simulink library "lib_ofdmrx"  (R2020a)
settings: Solver=VariableStepAuto  StartTime=0.0  StopTime=10.0  RelTol=1e-3
undefined symbols (not defined in the file): fs, LTSfreq, pilot, read_addr_rx, sc_index
libraries: simulink x36, hdlsllib x28, dspsigops x4, dsphdlmathfun x3, dsphdlxfrm x1, dsphdlsigops x1
(part 1 of 3)
settings Model: Creator=LDM  LastModifiedBy=LDM

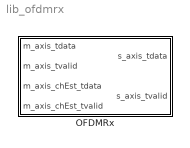
== system lib_ofdmrx ==
  OFDMRx : Subsystem  TreatAsAtomicUnit=on

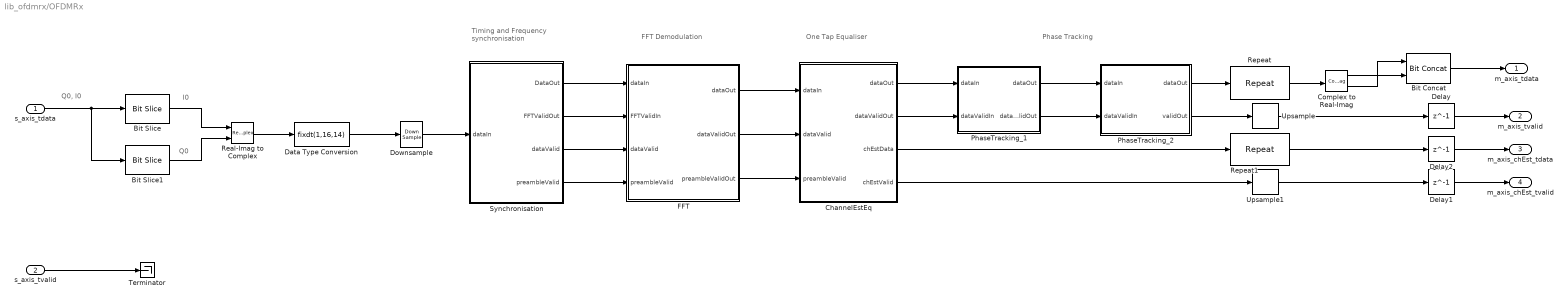
== system lib_ofdmrx/OFDMRx ==
  note: Q0
  note: I0
  note: Q0, I0
  note: Timing and Frequency
      | synchronisation
  note: FFT Demodulation
  note: One Tap Equaliser
  note: Phase Tracking
  s_axis_tdata : Inport
  s_axis_tvalid : Inport  Port=2
  Bit Concat : hdlsllib/Logic and Bit Operations/Bit Concat  numInputs=2
  Bit Slice : hdlsllib/Logic and Bit Operations/Bit Slice  lidx=15  ridx=0
      settings: SourceProductBaseCode=SL
  Bit Slice1 : hdlsllib/Logic and Bit Operations/Bit Slice  lidx=31  ridx=16
      settings: SourceProductBaseCode=SL
  ChannelEstEq : Subsystem
  Complex to Real-Imag : ComplexToRealImag
  Data Type Conversion : DataTypeConversion  OutDataTypeStr=fixdt(1,16,14)  ConvertRealWorld=Stored Integer (SI)
  Delay : Delay  DelayLength=1
  Delay1 : Delay  DelayLength=1
  Delay2 : Delay  DelayLength=1
  Downsample : DownSample  N=12  RateOptions=Allow multirate processing
  FFT : Subsystem
  PhaseTracking_1 : Subsystem
  PhaseTracking_2 : Subsystem
  Real-Imag to Complex : RealImagToComplex
  Repeat : dspsigops/Repeat  N=12  InputProcessing=Columns as channels (frame based)  RateOptions=Allow multirate processing  ic=0  mode=Unused parameter value
  Repeat1 : dspsigops/Repeat  N=12  InputProcessing=Columns as channels (frame based)  RateOptions=Allow multirate processing  ic=0  mode=Unused parameter value
  Synchronisation : Subsystem
  Terminator : Terminator
  Upsample : dspsigops/Upsample  N=12  phase=5  RateOptions=Allow multirate processing  ic=0  mode=Unused parameter value
  Upsample1 : dspsigops/Upsample  N=12  phase=5  RateOptions=Allow multirate processing  ic=0  mode=Unused parameter value
  m_axis_tdata : Outport  VectorParamsAs1DForOutWhenUnconnected=off
  m_axis_tvalid : Outport  Port=2  VectorParamsAs1DForOutWhenUnconnected=off
  m_axis_chEst_tdata : Outport  Port=3  VectorParamsAs1DForOutWhenUnconnected=off
  m_axis_chEst_tvalid : Outport  Port=4  VectorParamsAs1DForOutWhenUnconnected=off
  wires:
  Delay2/1 -> m_axis_chEst_tdata/1
  Repeat1/1 -> Delay2/1
  ChannelEstEq/3(chEstData) -> Repeat1/1
  ChannelEstEq/4(chEstValid) -> Upsample1/1
  Delay1/1 -> m_axis_chEst_tvalid/1
  Upsample1/1 -> Delay1/1
  PhaseTracking_1/2(dataValidOut) -> PhaseTracking_2/2(dataValidIn)
  PhaseTracking_1/1(dataOut) -> PhaseTracking_2/1(dataIn)
  ChannelEstEq/2(dataValidOut) -> PhaseTracking_1/2(dataValidIn)
  ChannelEstEq/1(dataOut) -> PhaseTracking_1/1(dataIn)
  Synchronisation/4(preambleValid) -> FFT/4(preambleValid)
  Synchronisation/3(dataValid) -> FFT/3(dataValid)
  Synchronisation/2(FFTValidOut) -> FFT/2(FFTValidIn)
  Synchronisation/1(DataOut) -> FFT/1(dataIn)
  FFT/2(dataValidOut) -> ChannelEstEq/2(dataValid)
  FFT/3(preambleValidOut) -> ChannelEstEq/3(preambleValid)
  FFT/1(dataOut) -> ChannelEstEq/1(dataIn)
  Real-Imag to Complex/1 -> Data Type Conversion/1
  Downsample/1 -> Synchronisation/1(dataIn)
  PhaseTracking_2/1(dataOut) -> Repeat/1
  PhaseTracking_2/2(validOut) -> Upsample/1
  Repeat/1 -> Complex to Real-Imag/1
  Complex to Real-Imag/2 -> Bit Concat/1
  Complex to Real-Imag/1 -> Bit Concat/2
  Bit Concat/1 -> m_axis_tdata/1
  Bit Slice/1 -> Real-Imag to Complex/1
  Bit Slice1/1 -> Real-Imag to Complex/2
  s_axis_tdata/1 -> Bit Slice1/1, Bit Slice/1
  s_axis_tvalid/1 -> Terminator/1
  Data Type Conversion/1 -> Downsample/1
  Upsample/1 -> Delay/1
  Delay/1 -> m_axis_tvalid/1

== system lib_ofdmrx/OFDMRx/ChannelEstEq ==
  dataIn : Inport
  dataValid : Inport  Port=2
  preambleValid : Inport  Port=3
  Bit Concat1 : hdlsllib/Logic and Bit Operations/Bit Concat  numInputs=2
  ChannelEstimate : Subsystem
  Complex to Real-Imag1 : ComplexToRealImag
  Data Type Conversion1 : DataTypeConversion  OutDataTypeStr=fixdt(1,16,14)
  Data Type Conversion3 : DataTypeConversion  OutDataTypeStr=uint16  ConvertRealWorld=Stored Integer (SI)
  Data Type Conversion4 : DataTypeConversion  OutDataTypeStr=uint16  ConvertRealWorld=Stored Integer (SI)
  Delay : Delay  DelayLength=6
  Equalise : Subsystem
  dataOut : Outport  VectorParamsAs1DForOutWhenUnconnected=off
  dataValidOut : Outport  Port=2  VectorParamsAs1DForOutWhenUnconnected=off
  chEstData : Outport  Port=3  VectorParamsAs1DForOutWhenUnconnected=off
  chEstValid : Outport  Port=4  VectorParamsAs1DForOutWhenUnconnected=off
  wires:
  Data Type Conversion1/1 -> Complex to Real-Imag1/1
  Complex to Real-Imag1/1 -> Data Type Conversion3/1
  Complex to Real-Imag1/2 -> Data Type Conversion4/1
  Data Type Conversion3/1 -> Bit Concat1/2
  Bit Concat1/1 -> chEstData/1
  Data Type Conversion4/1 -> Bit Concat1/1
  ChannelEstimate/2(dataValidOut) -> Equalise/3(dataValidIn), chEstValid/1
  Equalise/2(dataValidOut) -> dataValidOut/1
  Equalise/1(dataOutEq) -> dataOut/1
  dataValid/1 -> ChannelEstimate/3(dataValidIn)
  preambleValid/1 -> ChannelEstimate/2(preambleValid)
  dataIn/1 -> Delay/1, ChannelEstimate/1(dataIn)
  Delay/1 -> Equalise/1(dataInEq)
  ChannelEstimate/1(chEstOut) -> Data Type Conversion1/1, Equalise/2(chEstIn)

== system lib_ofdmrx/OFDMRx/FFT ==
  dataIn : Inport
  FFTValidIn : Inport  Port=2
  dataValid : Inport  Port=3
  preambleValid : Inport  Port=4
  Delay1 : Delay  DelayLength=173
  Delay2 : Delay  DelayLength=173
  FFT HDL Optimized : dsphdlxfrm/FFT HDL Optimized  FFTLength=64  Architecture=Streaming Radix 2^2  ComplexMultiplication=Use 4 multipliers and 2 adders  BitReversedOutput=off  BitReversedInput=off  Normalize=off  SimulateUsing=Code generation  RoundingMethod=Floor  ResetInputPort=off  StartOutputPort=off  EndOutputPort=off
      settings: SourceProductBaseCode=DS
  Terminator : Terminator
  dataOut : Outport  VectorParamsAs1DForOutWhenUnconnected=off
  dataValidOut : Outport  Port=2  VectorParamsAs1DForOutWhenUnconnected=off
  preambleValidOut : Outport  Port=3  VectorParamsAs1DForOutWhenUnconnected=off
  wires:
  preambleValid/1 -> Delay1/1
  dataValid/1 -> Delay2/1
  FFT HDL Optimized/2 -> Terminator/1
  FFT HDL Optimized/1 -> dataOut/1
  Delay1/1 -> preambleValidOut/1
  Delay2/1 -> dataValidOut/1
  dataIn/1 -> FFT HDL Optimized/1
  FFTValidIn/1 -> FFT HDL Optimized/2

== system lib_ofdmrx/OFDMRx/PhaseTracking_1 ==
  note: Phase Tracking Stage 1: Track linear phase error which occurs due to sampling phase/frequency offsets. The implemented algorithm
      | estimates the gradient of the linear phase error using pilot sub-carriers.
  dataIn : Inport
  dataValidIn : Inport  Port=2
  CordicRotate : Subsystem
  DataArrange : Subsystem
  "GradientEstimate " : Subsystem
  PhaseErrorEst : Subsystem
  PilotCtrlGen : Subsystem
  dataOut : Outport
  dataValidOut : Outport  Port=2
  wires:
  PilotCtrlGen/4(dataValid) -> "GradientEstimate "/4(dataValid)
  PilotCtrlGen/3(pilotEnd) -> "GradientEstimate "/3(PilotEnd)
  PilotCtrlGen/2(pilotOut) -> "GradientEstimate "/2(pilotIn)
  PilotCtrlGen/1(dataOut) -> "GradientEstimate "/1(dataIn)
  DataArrange/2(dataValidOut) -> PilotCtrlGen/2(validIn)
  DataArrange/1(dataOut) -> PilotCtrlGen/1(dataIn)
  dataValidIn/1 -> DataArrange/2(dataValidIn)
  dataIn/1 -> DataArrange/1(dataIn)
  CordicRotate/1("DataOutRotate  ") -> dataOut/1
  "GradientEstimate "/3(dataValidOut) -> PhaseErrorEst/3(dataValidIn)
  "GradientEstimate "/2(gradientOut) -> PhaseErrorEst/2(gradientIn)
  "GradientEstimate "/1(dataOut) -> PhaseErrorEst/1(dataIn)
  PhaseErrorEst/1(dataOut) -> CordicRotate/1(DataInRotate)
  PhaseErrorEst/2(PhaseOut) -> CordicRotate/2(PhaseInRotate)
  PhaseErrorEst/3(dataValidOut) -> CordicRotate/3(dataValidIn)
  CordicRotate/2(dataValidOut) -> dataValidOut/1

== system lib_ofdmrx/OFDMRx/PhaseTracking_2 ==
  note: Phase Tracking Stage 2:  Track Common Phase Error (CPE) from symbol to symbol.
      | CPE is caused by residual frequency offset and phase noise effects.
  dataIn : Inport
  dataValidIn : Inport  Port=2
  CordicRotate : Subsystem
  PhaseEst : Subsystem
  PilotCtrlGen : Subsystem
  dataOut : Outport  VectorParamsAs1DForOutWhenUnconnected=off
  validOut : Outport  Port=2  VectorParamsAs1DForOutWhenUnconnected=off
  wires:
  dataValidIn/1 -> PilotCtrlGen/2(ValidIn)
  dataIn/1 -> PilotCtrlGen/1(dataIn)
  CordicRotate/2(validOut) -> validOut/1
  CordicRotate/1("DataOut  ") -> dataOut/1
  PhaseEst/3(validOut) -> CordicRotate/3(validIn)
  PhaseEst/2(phaseOut) -> CordicRotate/2(PhaseIn)
  PhaseEst/1(dataOut) -> CordicRotate/1(DataIn)
  PilotCtrlGen/4(dataValid) -> PhaseEst/4(dataValid)
  PilotCtrlGen/3(PilotEnd) -> PhaseEst/3(pilotEnd)
  PilotCtrlGen/2(pilotOut) -> PhaseEst/2(PilotIn)
  PilotCtrlGen/1(dataOut) -> PhaseEst/1(dataIn)

== system lib_ofdmrx/OFDMRx/Synchronisation ==
  dataIn : Inport
  CoarseFreqCorr : Subsystem
  ControlSigGen : Subsystem
  Delay : Subsystem
  Delay1 : Delay  DelayLength=22  InputProcessing=Columns as channels (frame based)
  Delay2 : Delay  InputProcessing=Columns as channels (frame based)
  Delay4 : Delay  DelayLength=1  InputProcessing=Columns as channels (frame based)
  FrameDetect : Subsystem
  "SchmidlCoxMetric " : Subsystem
  DataOut : Outport  VectorParamsAs1DForOutWhenUnconnected=off
  FFTValidOut : Outport  Port=2  VectorParamsAs1DForOutWhenUnconnected=off
  dataValid : Outport  Port=3  VectorParamsAs1DForOutWhenUnconnected=off
  preambleValid : Outport  Port=4  VectorParamsAs1DForOutWhenUnconnected=off
  wires:
  Delay/1(dataOut) -> Delay4/1
  Delay/2(strobeOut) -> ControlSigGen/1(validIn)
  CoarseFreqCorr/1(dataOut) -> Delay/1(data)
  CoarseFreqCorr/2(frameDetOut) -> Delay/2(strobe)
  Delay4/1 -> DataOut/1
  FrameDetect/1(frameDet) -> CoarseFreqCorr/2(frameDet)
  Delay2/1 -> CoarseFreqCorr/1(dataIn)
  FrameDetect/2(phaseOut) -> CoarseFreqCorr/3(phaseIn)
  "SchmidlCoxMetric "/3(phase) -> FrameDetect/3(phaseIn)
  "SchmidlCoxMetric "/2(right) -> FrameDetect/2(rightIn)
  "SchmidlCoxMetric "/1(left) -> FrameDetect/1(leftIn)
  Delay1/1 -> Delay2/1
  ControlSigGen/3(preambleValid) -> preambleValid/1
  ControlSigGen/2(dataValid) -> dataValid/1
  ControlSigGen/1(FFTValid) -> FFTValidOut/1
  dataIn/1 -> Delay1/1, "SchmidlCoxMetric "/1(dataIn)

== system lib_ofdmrx/OFDMRx/ChannelEstEq/ChannelEstimate ==
  note: Get and store the channel estimate using the two
      | repetitions of the L-LTF
  note: Write averaged channel estimate to RAM and read out when data is valid
      | for equalisation of successive OFDM symbols.
  note: Note the preamble symbols do not pass this point.
  dataIn : Inport
  preambleValid : Inport  Port=2
  dataValidIn : Inport  Port=3
  ChanEst : Subsystem
  Delay : Delay  DelayLength=5
  Delay1 : Delay  DelayLength=5
  Delay2 : Delay  DelayLength=1
  Dual Port RAM1 : hdlsllib/HDL RAMs/Dual Port RAM  ram_size=6
      settings: SourceProductBaseCode=SL
  HDL Counter3 : hdlsllib/Sources/HDL Counter  CountType=Count limited  CountInit=0  CountStep=1  CountMax=63  CountFromType=Initial value  CountFrom=0  CountResetPort=off  CountLoadPort=off  CountEnbPort=on  CountDirPort=off  CountDataType=Unsigned  CountWordLen=6  CountFracLen=0  CountSampTime=1
  Terminator : Terminator
  WriteEnbAddrGen : Subsystem
  chEstOut : Outport  VectorParamsAs1DForOutWhenUnconnected=off
  dataValidOut : Outport  Port=2  VectorParamsAs1DForOutWhenUnconnected=off
  wires:
  Dual Port RAM1/1 -> Terminator/1
  WriteEnbAddrGen/2(Out2) -> Dual Port RAM1/3
  WriteEnbAddrGen/1(Out1) -> Dual Port RAM1/2
  Delay/1 -> WriteEnbAddrGen/1(In1)
  Delay1/1 -> Delay2/1, HDL Counter3/1
  dataValidIn/1 -> Delay1/1
  ChanEst/1(ChEstOut) -> Dual Port RAM1/1
  dataIn/1 -> ChanEst/1(ChanEstIn)
  preambleValid/1 -> Delay/1, ChanEst/2(PreambValidIn)
  Delay2/1 -> dataValidOut/1
  Dual Port RAM1/2 -> chEstOut/1
  HDL Counter3/1 -> Dual Port RAM1/4

== system lib_ofdmrx/OFDMRx/ChannelEstEq/Equalise ==
  note: Perform a complex division to obtain equalised data symbols.
  dataInEq : Inport
  chEstIn : Inport  Port=2
  dataValidIn : Inport  Port=3
  Abs2 : Subsystem
  Complex Mult : Subsystem
  Delay1 : Delay
  Delay8 : Delay  DelayLength=3
  Divide : Subsystem
  dataOutEq : Outport  VectorParamsAs1DForOutWhenUnconnected=off
  dataValidOut : Outport  Port=2  VectorParamsAs1DForOutWhenUnconnected=off
  wires:
  Divide/1(dataOutEq) -> dataOutEq/1
  Delay1/1 -> dataValidOut/1
  Delay8/1 -> Delay1/1
  Abs2/1(Out1) -> Divide/2(In2)
  Complex Mult/1(Out1) -> Divide/1(In1)
  dataInEq/1 -> Complex Mult/1(In1)
  chEstIn/1 -> Complex Mult/2(In2), Abs2/1(ChEstIn)
  dataValidIn/1 -> Delay8/1

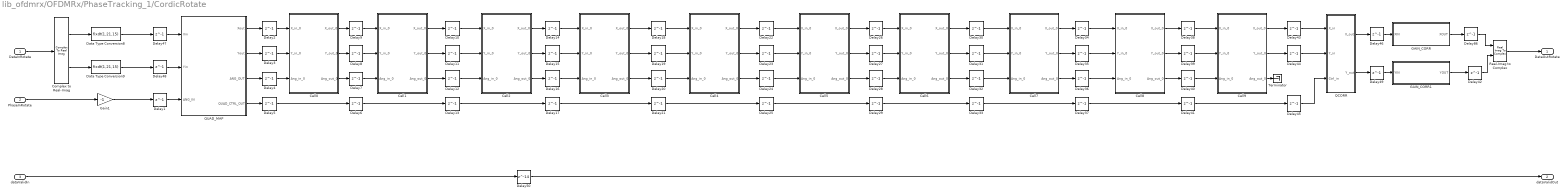
== system lib_ofdmrx/OFDMRx/PhaseTracking_1/CordicRotate ==
  DataInRotate : Inport
  PhaseInRotate : Inport  Port=2
  dataValidIn : Inport  Port=3
  Cell0 : Subsystem
  Cell1 : Subsystem
  Cell2 : Subsystem
  Cell3 : Subsystem
  Cell4 : Subsystem
  Cell5 : Subsystem
  Cell6 : Subsystem
  Cell7 : Subsystem
  Cell8 : Subsystem
  Cell9 : Subsystem
  Complex to Real-Imag : ComplexToRealImag
  Data Type Conversion8 : DataTypeConversion  OutDataTypeStr=fixdt(1,21,15)
  Data Type Conversion9 : DataTypeConversion  OutDataTypeStr=fixdt(1,21,15)
  Delay{1..49,86} (50 alike) : Delay  DelayLength=1
  Delay50 : Delay  DelayLength=14
  GAIN_CORR : Subsystem
  GAIN_CORR1 : Subsystem
  Gain1 : Gain  Gain=-1  OutDataTypeStr=fixdt(1,23,20)
  QCORR : Subsystem
  QUAD_MAP : Subsystem
  Real-Imag to Complex : RealImagToComplex
  Terminator : Terminator
  "DataOutRotate  " : Outport  VectorParamsAs1DForOutWhenUnconnected=off
  dataValidOut : Outport  Port=2  VectorParamsAs1DForOutWhenUnconnected=off
  wires:
  Real-Imag to Complex/1 -> "DataOutRotate  "/1
  Delay42/1 -> Real-Imag to Complex/2
  Delay86/1 -> Real-Imag to Complex/1
  Complex to Real-Imag/1 -> Data Type Conversion8/1
  DataInRotate/1 -> Complex to Real-Imag/1
  Complex to Real-Imag/2 -> Data Type Conversion9/1
  GAIN_CORR/1(XOUT) -> Delay86/1
  Delay48/1 -> QUAD_MAP/2(Yin)
  Delay47/1 -> QUAD_MAP/1(Xin)
  QUAD_MAP/1(Xout) -> Delay2/1
  QUAD_MAP/2(Yout) -> Delay3/1
  QUAD_MAP/3(ANG_OUT) -> Delay4/1
  Delay2/1 -> Cell0/1(X_in_0)
  Delay3/1 -> Cell0/2(Y_in_0)
  QUAD_MAP/4(QUAD_CTRL_OUT) -> Delay5/1
  Cell0/1(X_out_0) -> Delay9/1
  Cell0/2(Y_out_0) -> Delay8/1
  Cell0/3(Ang_out_0) -> Delay7/1
  Delay5/1 -> Delay6/1
  Delay7/1 -> Cell1/3(Ang_in_0)
  Delay8/1 -> Cell1/2(Y_in_0)
  Delay9/1 -> Cell1/1(X_in_0)
  Cell1/1(X_out_0) -> Delay10/1
  Cell1/2(Y_out_0) -> Delay11/1
  Cell1/3(Ang_out_0) -> Delay12/1
  Delay6/1 -> Delay13/1
  Delay10/1 -> Cell2/1(X_in_0)
  Delay11/1 -> Cell2/2(Y_in_0)
  Delay12/1 -> Cell2/3(Ang_in_0)
  Delay16/1 -> Cell3/3(Ang_in_0)
  Delay15/1 -> Cell3/2(Y_in_0)
  Delay14/1 -> Cell3/1(X_in_0)
  Delay13/1 -> Delay17/1
  Cell2/3(Ang_out_0) -> Delay16/1
  Cell2/2(Y_out_0) -> Delay15/1
  Cell2/1(X_out_0) -> Delay14/1
  Cell3/1(X_out_0) -> Delay18/1
  Cell3/2(Y_out_0) -> Delay19/1
  Cell3/3(Ang_out_0) -> Delay20/1
  Delay17/1 -> Delay21/1
  Delay18/1 -> Cell4/1(X_in_0)
  Delay19/1 -> Cell4/2(Y_in_0)
  Delay20/1 -> Cell4/3(Ang_in_0)
  Delay24/1 -> Cell5/3(Ang_in_0)
  Delay23/1 -> Cell5/2(Y_in_0)
  Delay22/1 -> Cell5/1(X_in_0)
  Delay21/1 -> Delay25/1
  Cell4/3(Ang_out_0) -> Delay24/1
  Cell4/2(Y_out_0) -> Delay23/1
  Cell4/1(X_out_0) -> Delay22/1
  Cell5/1(X_out_0) -> Delay26/1
  Cell5/2(Y_out_0) -> Delay27/1
  Cell5/3(Ang_out_0) -> Delay28/1
  Delay25/1 -> Delay29/1
  Delay26/1 -> Cell6/1(X_in_0)
  Delay27/1 -> Cell6/2(Y_in_0)
  Delay28/1 -> Cell6/3(Ang_in_0)
  Delay32/1 -> Cell7/3(Ang_in_0)
  Delay31/1 -> Cell7/2(Y_in_0)
  Delay30/1 -> Cell7/1(X_in_0)
  Delay29/1 -> Delay33/1
  Cell6/3(Ang_out_0) -> Delay32/1
  Cell6/2(Y_out_0) -> Delay31/1
  Cell6/1(X_out_0) -> Delay30/1
  Cell7/1(X_out_0) -> Delay34/1
  Cell7/2(Y_out_0) -> Delay35/1
  Cell7/3(Ang_out_0) -> Delay36/1
  Delay33/1 -> Delay37/1
  Delay34/1 -> Cell8/1(X_in_0)
  Delay35/1 -> Cell8/2(Y_in_0)
  Delay36/1 -> Cell8/3(Ang_in_0)
  Delay40/1 -> Cell9/3(Ang_in_0)
  Delay39/1 -> Cell9/2(Y_in_0)
  Delay38/1 -> Cell9/1(X_in_0)
  Delay37/1 -> Delay41/1
  Cell8/3(Ang_out_0) -> Delay40/1
  Cell8/2(Y_out_0) -> Delay39/1
  Cell8/1(X_out_0) -> Delay38/1
  GAIN_CORR1/1(YOUT) -> Delay42/1
  Cell9/3(Ang_out_0) -> Terminator/1
  Delay41/1 -> Delay45/1
  Cell9/1(X_out_0) -> Delay43/1
  Cell9/2(Y_out_0) -> Delay44/1
  Delay43/1 -> QCORR/1(X_in)
  Delay44/1 -> QCORR/2(Y_in)
  Delay46/1 -> GAIN_CORR/1(XIN)
  Delay49/1 -> GAIN_CORR1/1(YIN)
  QCORR/2(Y_out) -> Delay49/1
  Delay1/1 -> QUAD_MAP/3(ANG_IN)
  Delay4/1 -> Cell0/3(Ang_in_0)
  Delay45/1 -> QCORR/3(Ctrl_in)
  Data Type Conversion8/1 -> Delay47/1
  Data Type Conversion9/1 -> Delay48/1
  QCORR/1(X_out) -> Delay46/1
  PhaseInRotate/1 -> Gain1/1
  Gain1/1 -> Delay1/1
  dataValidIn/1 -> Delay50/1
  Delay50/1 -> dataValidOut/1

== system lib_ofdmrx/OFDMRx/PhaseTracking_1/DataArrange ==
  note: Re-arrange data symbols
  dataIn : Inport
  dataValidIn : Inport  Port=2
  Delay : Delay  DelayLength=64  InitialCondition=0  UseCircularBuffer=on
  Delay3 : Delay  DelayLength=1  InitialCondition=0  UseCircularBuffer=on
  Dual Port RAM : hdlsllib/HDL RAMs/Dual Port RAM  ram_size=7
      settings: SourceProductBaseCode=SL
  HDL Counter : hdlsllib/Sources/HDL Counter  CountType=Count limited  CountInit=0  CountStep=1  CountMax=127  CountFromType=Initial value  CountFrom=0  CountResetPort=off  CountLoadPort=off  CountEnbPort=on  CountDirPort=off  CountDataType=Unsigned  CountWordLen=7  CountFracLen=0  CountSampTime=1
  HDL Counter1 : hdlsllib/Sources/HDL Counter  CountType=Count limited  CountInit=0  CountStep=1  CountMax=127  CountFromType=Initial value  CountFrom=0  CountResetPort=off  CountLoadPort=off  CountEnbPort=on  CountDirPort=off  CountDataType=Unsigned  CountWordLen=7  CountFracLen=0  CountSampTime=1
  READ_ADDRESS : Lookup_n-D  NumberOfTableDimensions=1  LookupTableObject=''  BreakpointsForDimension1=[0:127]  BreakpointsForDimension1FirstPoint=10  BreakpointsForDimension2FirstPoint=10  BreakpointsForDimension1Spacing=12  BreakpointsForDimension2Spacing=12  IndexSearchMethod=Evenly spaced points  Table=read_addr_rx  TableDataTypeStr=fixdt(0,7,0)  InterpMethod=Flat  DiagnosticForOutOfRangeInput=Error  InternalRulePriority=Speed  OutDataTypeStr=fixdt(0,7,0)  RndMeth=Simplest  InputSameDT=on
  READ_CTRL : Subsystem
  Terminator : Terminator
  dataValidGen : Subsystem
  dataOut : Outport  VectorParamsAs1DForOutWhenUnconnected=off
  dataValidOut : Outport  Port=2  VectorParamsAs1DForOutWhenUnconnected=off
  wires:
  dataValidGen/1(dataValidOut) -> dataValidOut/1
  Delay3/1 -> dataValidGen/1(enb)
  READ_ADDRESS/1 -> READ_CTRL/1(In1)
  READ_CTRL/1(Out1) -> Dual Port RAM/4
  Delay/1 -> READ_CTRL/2(In2), Delay3/1, HDL Counter/1
  HDL Counter1/1 -> Dual Port RAM/2
  dataIn/1 -> Dual Port RAM/1
  Dual Port RAM/2 -> dataOut/1
  HDL Counter/1 -> READ_ADDRESS/1
  dataValidIn/1 -> Dual Port RAM/3, HDL Counter1/1, Delay/1
  Dual Port RAM/1 -> Terminator/1

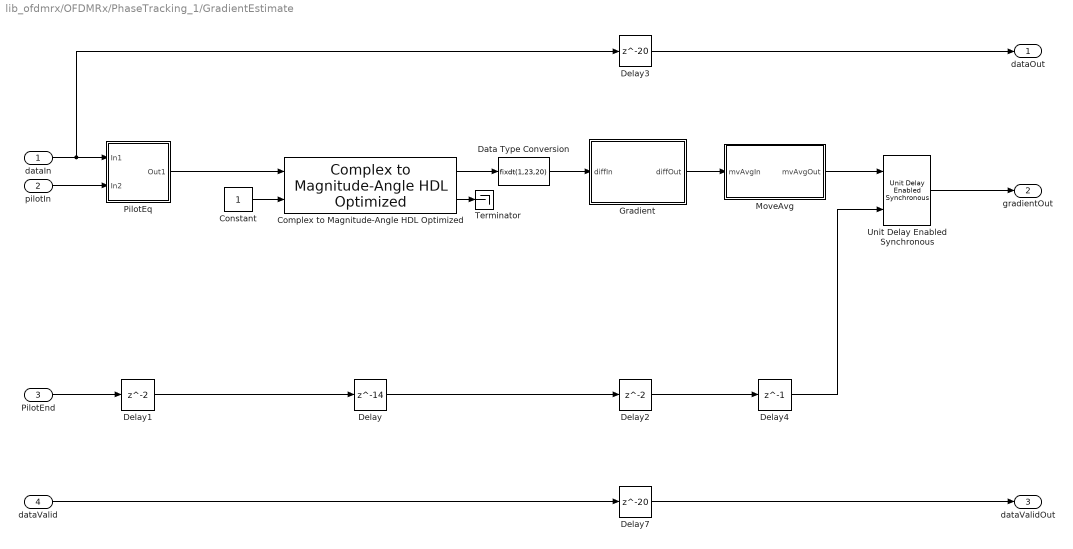
== system lib_ofdmrx/OFDMRx/PhaseTracking_1/GradientEstimate  ==
  dataIn : Inport
  pilotIn : Inport  Port=2
  PilotEnd : Inport  Port=3
  dataValid : Inport  Port=4
  Complex to Magnitude-Angle HDL Optimized : dsphdlmathfun/Complex to Magnitude-Angle HDL Optimized  NumIterationsSource=Property  NumIterations=10  OutputFormat=Angle  AngleFormat=Radians  ScaleOutput=off  SimulateUsing=Code generation
      settings: SourceProductBaseCode=DS
  Constant : Constant  OutDataTypeStr=boolean  SampleTime=1/fs
  Data Type Conversion : DataTypeConversion  OutDataTypeStr=fixdt(1,23,20)
  Delay : Delay  DelayLength=14
  Delay1 : Delay
  Delay2 : Delay
  Delay3 : Delay  DelayLength=20
  Delay4 : Delay  DelayLength=1
  Delay7 : Delay  DelayLength=20
  Gradient : Subsystem
  MoveAvg : Subsystem
  PilotEq : Subsystem
  Terminator : Terminator
  Unit Delay Enabled Synchronous : hdlsllib/Discrete/Unit Delay Enabled Synchronous  InitialCondition=0.0  SampleTime=-1
      settings: SourceProductBaseCode=SL
  dataOut : Outport  VectorParamsAs1DForOutWhenUnconnected=off
  gradientOut : Outport  Port=2  VectorParamsAs1DForOutWhenUnconnected=off
  dataValidOut : Outport  Port=3  VectorParamsAs1DForOutWhenUnconnected=off
  wires:
  Delay4/1 -> Unit Delay Enabled Synchronous/2
  Delay/1 -> Delay2/1
  PilotEnd/1 -> Delay1/1
  dataValid/1 -> Delay7/1
  Gradient/1(diffOut) -> MoveAvg/1(mvAvgIn)
  dataIn/1 -> Delay3/1, PilotEq/1(In1)
  pilotIn/1 -> PilotEq/2(In2)
  PilotEq/1(Out1) -> Complex to Magnitude-Angle HDL Optimized/1
  Delay1/1 -> Delay/1
  MoveAvg/1(mvAvgOut) -> Unit Delay Enabled Synchronous/1
  Delay3/1 -> dataOut/1
  Unit Delay Enabled Synchronous/1 -> gradientOut/1
  Delay7/1 -> dataValidOut/1
  Complex to Magnitude-Angle HDL Optimized/1 -> Data Type Conversion/1
  Constant/1 -> Complex to Magnitude-Angle HDL Optimized/2
  Complex to Magnitude-Angle HDL Optimized/2 -> Terminator/1
  Data Type Conversion/1 -> Gradient/1(diffIn)
  Delay2/1 -> Delay4/1

== system lib_ofdmrx/OFDMRx/PhaseTracking_1/PhaseErrorEst ==
  dataIn : Inport
  gradientIn : Inport  Port=2
  dataValidIn : Inport  Port=3
  Delay{2..8} (7 alike) : Delay  DelayLength=1
  HDL Counter : hdlsllib/Sources/HDL Counter  CountType=Count limited  CountInit=0  CountStep=1  CountMax=51  CountFromType=Initial value  CountFrom=0  CountResetPort=on  CountLoadPort=off  CountEnbPort=on  CountDirPort=off  CountDataType=Unsigned  CountWordLen=6  CountFracLen=0  CountSampTime=1
  LUT : Lookup_n-D  NumberOfTableDimensions=1  BreakpointsForDimension1=0:51  IndexSearchMethod=Evenly spaced points  Table=sc_index  TableDataTypeStr=fixdt(1,6,0)  InterpMethod=Flat  ExtrapMethod=Clip  DiagnosticForOutOfRangeInput=Error  UseLastTableValue=on  InternalRulePriority=Speed  OutDataTypeStr=fixdt(1,6,0)  RndMeth=Simplest  InputSameDT=on
  NOT : Logic  Operator=NOT  IconShape=distinctive  AllPortsSameDT=off  OutDataTypeStr=boolean
  Product : Product  OutDataTypeStr=fixdt(1,23,20)
  dataOut : Outport  VectorParamsAs1DForOutWhenUnconnected=off
  PhaseOut : Outport  Port=2  VectorParamsAs1DForOutWhenUnconnected=off
  dataValidOut : Outport  Port=3  VectorParamsAs1DForOutWhenUnconnected=off
  wires:
  dataValidIn/1 -> NOT/1, Delay4/1, HDL Counter/2
  dataIn/1 -> Delay2/1
  gradientIn/1 -> Delay3/1
  LUT/1 -> Delay5/1
  NOT/1 -> HDL Counter/1
  HDL Counter/1 -> LUT/1
  Delay3/1 -> Product/1
  Delay5/1 -> Product/2
  Delay2/1 -> Delay6/1
  Delay6/1 -> dataOut/1
  Product/1 -> Delay7/1
  Delay7/1 -> PhaseOut/1
  Delay4/1 -> Delay8/1
  Delay8/1 -> dataValidOut/1

== system lib_ofdmrx/OFDMRx/PhaseTracking_1/PilotCtrlGen ==
  dataIn : Inport
  validIn : Inport  Port=2
  CtrlSigGen : Subsystem
  Delay1 : Delay  DelayLength=1
  Delay10 : Delay  DelayLength=1
  SampleCounter : Subsystem
  SymbolCounter : Subsystem
  pilotGen : Subsystem
  dataOut : Outport  VectorParamsAs1DForOutWhenUnconnected=off
  pilotOut : Outport  Port=2  VectorParamsAs1DForOutWhenUnconnected=off
  pilotEnd : Outport  Port=3  VectorParamsAs1DForOutWhenUnconnected=off
  dataValid : Outport  Port=4  VectorParamsAs1DForOutWhenUnconnected=off
  wires:
  Delay1/1 -> pilotGen/3(valid), CtrlSigGen/1(valid)
  SampleCounter/1(Sample_Cnt) -> pilotGen/2(sampleCount), CtrlSigGen/2(sampleCount)
  CtrlSigGen/2(pilotEnd) -> pilotEnd/1
  CtrlSigGen/1(dataValid) -> dataValid/1
  SymbolCounter/1(Symbl_cnt) -> pilotGen/1(symbCount)
  validIn/1 -> Delay1/1, SampleCounter/1(Valid_In), SymbolCounter/1(ValidIn)
  pilotGen/1(pilOut) -> pilotOut/1
  Delay10/1 -> dataOut/1
  dataIn/1 -> Delay10/1

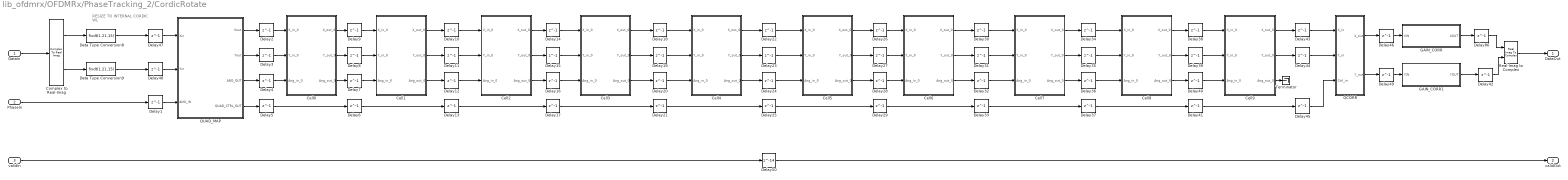
== system lib_ofdmrx/OFDMRx/PhaseTracking_2/CordicRotate ==
  note: RESIZE TO INTERNAL
      | CORDIC WL
  DataIn : Inport
  PhaseIn : Inport  Port=2
  validIn : Inport  Port=3
  Cell0 : Subsystem
  Cell1 : Subsystem
  Cell2 : Subsystem
  Cell3 : Subsystem
  Cell4 : Subsystem
  Cell5 : Subsystem
  Cell6 : Subsystem
  Cell7 : Subsystem
  Cell8 : Subsystem
  Cell9 : Subsystem
  Complex to Real-Imag : ComplexToRealImag
  Data Type Conversion8 : DataTypeConversion  OutDataTypeStr=fixdt(1,21,15)
  Data Type Conversion9 : DataTypeConversion  OutDataTypeStr=fixdt(1,21,15)
  Delay{1..49,86} (50 alike) : Delay  DelayLength=1
  Delay50 : Delay  DelayLength=14
  GAIN_CORR : Subsystem
  GAIN_CORR1 : Subsystem
  QCORR : Subsystem
  QUAD_MAP : Subsystem
  Real-Imag to Complex : RealImagToComplex
  Terminator : Terminator
  "DataOut  " : Outport  VectorParamsAs1DForOutWhenUnconnected=off
  validOut : Outport  Port=2  VectorParamsAs1DForOutWhenUnconnected=off
  wires:
  Delay50/1 -> validOut/1
  validIn/1 -> Delay50/1
  Real-Imag to Complex/1 -> "DataOut  "/1
  Delay42/1 -> Real-Imag to Complex/2
  Delay86/1 -> Real-Imag to Complex/1
  Complex to Real-Imag/1 -> Data Type Conversion8/1
  DataIn/1 -> Complex to Real-Imag/1
  Complex to Real-Imag/2 -> Data Type Conversion9/1
  GAIN_CORR/1(XOUT) -> Delay86/1
  Delay48/1 -> QUAD_MAP/2(Yin)
  Delay47/1 -> QUAD_MAP/1(Xin)
  QUAD_MAP/1(Xout) -> Delay2/1
  QUAD_MAP/2(Yout) -> Delay3/1
  QUAD_MAP/3(ANG_OUT) -> Delay4/1
  Delay2/1 -> Cell0/1(X_in_0)
  Delay3/1 -> Cell0/2(Y_in_0)
  QUAD_MAP/4(QUAD_CTRL_OUT) -> Delay5/1
  Cell0/1(X_out_0) -> Delay9/1
  Cell0/2(Y_out_0) -> Delay8/1
  Cell0/3(Ang_out_0) -> Delay7/1
  Delay5/1 -> Delay6/1
  Delay7/1 -> Cell1/3(Ang_in_0)
  Delay8/1 -> Cell1/2(Y_in_0)
  Delay9/1 -> Cell1/1(X_in_0)
  Cell1/1(X_out_0) -> Delay10/1
  Cell1/2(Y_out_0) -> Delay11/1
  Cell1/3(Ang_out_0) -> Delay12/1
  Delay6/1 -> Delay13/1
  Delay10/1 -> Cell2/1(X_in_0)
  Delay11/1 -> Cell2/2(Y_in_0)
  Delay12/1 -> Cell2/3(Ang_in_0)
  Delay16/1 -> Cell3/3(Ang_in_0)
  Delay15/1 -> Cell3/2(Y_in_0)
  Delay14/1 -> Cell3/1(X_in_0)
  Delay13/1 -> Delay17/1
  Cell2/3(Ang_out_0) -> Delay16/1
  Cell2/2(Y_out_0) -> Delay15/1
  Cell2/1(X_out_0) -> Delay14/1
  Cell3/1(X_out_0) -> Delay18/1
  Cell3/2(Y_out_0) -> Delay19/1
  Cell3/3(Ang_out_0) -> Delay20/1
  Delay17/1 -> Delay21/1
  Delay18/1 -> Cell4/1(X_in_0)
  Delay19/1 -> Cell4/2(Y_in_0)
  Delay20/1 -> Cell4/3(Ang_in_0)
  Delay24/1 -> Cell5/3(Ang_in_0)
  Delay23/1 -> Cell5/2(Y_in_0)
  Delay22/1 -> Cell5/1(X_in_0)
  Delay21/1 -> Delay25/1
  Cell4/3(Ang_out_0) -> Delay24/1
  Cell4/2(Y_out_0) -> Delay23/1
  Cell4/1(X_out_0) -> Delay22/1
  Cell5/1(X_out_0) -> Delay26/1
  Cell5/2(Y_out_0) -> Delay27/1
  Cell5/3(Ang_out_0) -> Delay28/1
  Delay25/1 -> Delay29/1
  Delay26/1 -> Cell6/1(X_in_0)
  Delay27/1 -> Cell6/2(Y_in_0)
  Delay28/1 -> Cell6/3(Ang_in_0)
  Delay32/1 -> Cell7/3(Ang_in_0)
  Delay31/1 -> Cell7/2(Y_in_0)
  Delay30/1 -> Cell7/1(X_in_0)
  Delay29/1 -> Delay33/1
  Cell6/3(Ang_out_0) -> Delay32/1
  Cell6/2(Y_out_0) -> Delay31/1
  Cell6/1(X_out_0) -> Delay30/1
  Cell7/1(X_out_0) -> Delay34/1
  Cell7/2(Y_out_0) -> Delay35/1
  Cell7/3(Ang_out_0) -> Delay36/1
  Delay33/1 -> Delay37/1
  Delay34/1 -> Cell8/1(X_in_0)
  Delay35/1 -> Cell8/2(Y_in_0)
  Delay36/1 -> Cell8/3(Ang_in_0)
  Delay40/1 -> Cell9/3(Ang_in_0)
  Delay39/1 -> Cell9/2(Y_in_0)
  Delay38/1 -> Cell9/1(X_in_0)
  Delay37/1 -> Delay41/1
  Cell8/3(Ang_out_0) -> Delay40/1
  Cell8/2(Y_out_0) -> Delay39/1
  Cell8/1(X_out_0) -> Delay38/1
  GAIN_CORR1/1(YOUT) -> Delay42/1
  Cell9/3(Ang_out_0) -> Terminator/1
  Delay41/1 -> Delay45/1
  Cell9/1(X_out_0) -> Delay43/1
  Cell9/2(Y_out_0) -> Delay44/1
  Delay43/1 -> QCORR/1(X_in)
  Delay44/1 -> QCORR/2(Y_in)
  Delay46/1 -> GAIN_CORR/1(XIN)
  Delay49/1 -> GAIN_CORR1/1(YIN)
  QCORR/2(Y_out) -> Delay49/1
  Delay1/1 -> QUAD_MAP/3(ANG_IN)
  Delay4/1 -> Cell0/3(Ang_in_0)
  Delay45/1 -> QCORR/3(Ctrl_in)
  Data Type Conversion8/1 -> Delay47/1
  Data Type Conversion9/1 -> Delay48/1
  PhaseIn/1 -> Delay1/1
  QCORR/1(X_out) -> Delay46/1

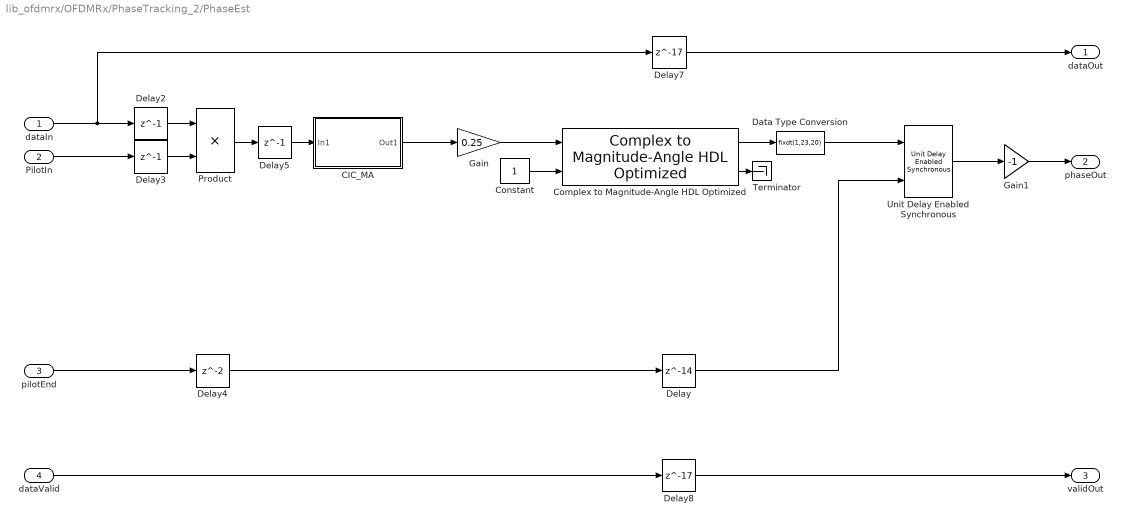
== system lib_ofdmrx/OFDMRx/PhaseTracking_2/PhaseEst ==
  dataIn : Inport
  PilotIn : Inport  Port=2
  pilotEnd : Inport  Port=3
  dataValid : Inport  Port=4
  CIC_MA : Subsystem
  Complex to Magnitude-Angle HDL Optimized : dsphdlmathfun/Complex to Magnitude-Angle HDL Optimized  NumIterationsSource=Property  NumIterations=10  OutputFormat=Angle  AngleFormat=Radians  ScaleOutput=off  SimulateUsing=Code generation
      settings: SourceProductBaseCode=DS
  Constant : Constant  OutDataTypeStr=boolean  SampleTime=1/fs
  Data Type Conversion : DataTypeConversion  OutDataTypeStr=fixdt(1,23,20)
  Delay : Delay  DelayLength=14
  Delay2 : Delay  DelayLength=1
  Delay3 : Delay  DelayLength=1
  Delay4 : Delay
  Delay5 : Delay  DelayLength=1
  Delay7 : Delay  DelayLength=17
  Delay8 : Delay  DelayLength=17
  Gain : Gain  Gain=0.25  OutDataTypeStr=fixdt(1,18,15)
  Gain1 : Gain  Gain=-1  OutDataTypeStr=fixdt(1,23,20)
  Product : Product  OutDataTypeStr=fixdt(1,18,15)
  Terminator : Terminator
  Unit Delay Enabled Synchronous : hdlsllib/Discrete/Unit Delay Enabled Synchronous  InitialCondition=0.0  SampleTime=-1
      settings: SourceProductBaseCode=SL
  dataOut : Outport  VectorParamsAs1DForOutWhenUnconnected=off
  phaseOut : Outport  Port=2  VectorParamsAs1DForOutWhenUnconnected=off
  validOut : Outport  Port=3  VectorParamsAs1DForOutWhenUnconnected=off
  wires:
  Data Type Conversion/1 -> Unit Delay Enabled Synchronous/1
  Gain1/1 -> phaseOut/1
  Delay4/1 -> Delay/1
  Complex to Magnitude-Angle HDL Optimized/2 -> Terminator/1
  Complex to Magnitude-Angle HDL Optimized/1 -> Data Type Conversion/1
  Gain/1 -> Complex to Magnitude-Angle HDL Optimized/1
  Constant/1 -> Complex to Magnitude-Angle HDL Optimized/2
  Delay8/1 -> validOut/1
  Unit Delay Enabled Synchronous/1 -> Gain1/1
  Delay7/1 -> dataOut/1
  dataValid/1 -> Delay8/1
  pilotEnd/1 -> Delay4/1
  Delay5/1 -> CIC_MA/1(In1)
  Delay3/1 -> Product/2
  Delay2/1 -> Product/1
  Product/1 -> Delay5/1
  dataIn/1 -> Delay2/1, Delay7/1
  PilotIn/1 -> Delay3/1
  Delay/1 -> Unit Delay Enabled Synchronous/2
  CIC_MA/1(Out1) -> Gain/1

== system lib_ofdmrx/OFDMRx/PhaseTracking_2/PilotCtrlGen ==
  dataIn : Inport
  ValidIn : Inport  Port=2
  CtrlSigGen : Subsystem
  Delay1 : Delay  DelayLength=1
  Delay10 : Delay  DelayLength=1
  SampleCounter : Subsystem
  SymbolCounter : Subsystem
  pilotGen : Subsystem
  dataOut : Outport  VectorParamsAs1DForOutWhenUnconnected=off
  pilotOut : Outport  Port=2  VectorParamsAs1DForOutWhenUnconnected=off
  PilotEnd : Outport  Port=3  VectorParamsAs1DForOutWhenUnconnected=off
  dataValid : Outport  Port=4  VectorParamsAs1DForOutWhenUnconnected=off
  wires:
  Delay1/1 -> pilotGen/3(valid), CtrlSigGen/1(valid)
  SampleCounter/1(Sample_Cnt) -> pilotGen/2(sampleCount), CtrlSigGen/2(sampleCount)
  CtrlSigGen/2(pilotEnd) -> PilotEnd/1
  CtrlSigGen/1(dataValid) -> dataValid/1
  SymbolCounter/1(Symbl_cnt) -> pilotGen/1(symbCount)
  ValidIn/1 -> SymbolCounter/1(ValidIn), SampleCounter/1(Valid_In), Delay1/1
  pilotGen/1(pilOut) -> pilotOut/1
  Delay10/1 -> dataOut/1
  dataIn/1 -> Delay10/1

== system lib_ofdmrx/OFDMRx/Synchronisation/CoarseFreqCorr ==
  note: Reccord the phase of the averaged autocorrelation at the coarse
      | timing point.
  note: Correct frequency offset
  note: Generate complex sinusoid with a frequency equal
      | to the estimated frequency offset.
  dataIn : Inport
  frameDet : Inport  Port=2
  phaseIn : Inport  Port=3
  Constant : Constant  VectorParams1D=off  OutDataTypeStr=boolean  SampleTime=1/fs
  Delay{,2,5,7} (4 alike) : Delay  DelayLength=1
  Delay1 : Delay  DelayLength=9
  Delay3 : Delay  DelayLength=6
  Gain : Gain  Gain=2048  OutDataTypeStr=uint16
  Math Function : Math  Operator=conj  SignedPower=on  RndMeth=Zero  SaturateOnIntegerOverflow=on
  NCO HDL Optimized : dsphdlsigops/NCO HDL Optimized  PhaseIncrementSource=Input port  PhaseIncrement=100  PhaseOffsetSource=Property  PhaseOffset=0  DitherSource=Property  NumDitherBits=4  SamplesPerFrame=1  LUTCompress=on  ResetAction=off  Waveform=Complex exponential  PhasePort=off  SimulateUsing=Code generation  AccumulatorWL=16  PhaseQuantization=on  NumQuantizerAccumulatorBits=12  OutputDataType=Binary point scaling  OutputWL=16  OutputFL=14
      settings: SourceProductBaseCode=DS
  Product : Product  OutDataTypeStr=fixdt(1,16,14)
  RsingEdge : Subsystem
  Terminator : Terminator
  Unit Delay Enabled Synchronous : hdlsllib/Discrete/Unit Delay Enabled Synchronous  InitialCondition=0.0  SampleTime=-1
      settings: SourceProductBaseCode=SL
  dataOut : Outport  VectorParamsAs1DForOutWhenUnconnected=off
  frameDetOut : Outport  Port=2  VectorParamsAs1DForOutWhenUnconnected=off
  wires:
  Delay7/1 -> dataOut/1
  Delay1/1 -> frameDetOut/1
  Math Function/1 -> Delay5/1
  Delay3/1 -> Delay/1
  Product/1 -> Delay7/1
  Delay5/1 -> Product/2
  Delay/1 -> Product/1
  dataIn/1 -> Delay2/1
  phaseIn/1 -> Unit Delay Enabled Synchronous/1
  RsingEdge/1(Out1) -> Unit Delay Enabled Synchronous/2
  frameDet/1 -> Delay1/1, RsingEdge/1(In1)
  Delay2/1 -> Delay3/1
  Unit Delay Enabled Synchronous/1 -> Gain/1
  Gain/1 -> NCO HDL Optimized/1
  NCO HDL Optimized/1 -> Math Function/1
  NCO HDL Optimized/2 -> Terminator/1
  Constant/1 -> NCO HDL Optimized/2

== system lib_ofdmrx/OFDMRx/Synchronisation/ControlSigGen ==
  validIn : Inport
  OR : Logic  Operator=OR  IconShape=distinctive  AllPortsSameDT=off  OutDataTypeStr=boolean
  PreambleValidGen : Subsystem
  dataValidGen : Subsystem
  FFTValid : Outport  VectorParamsAs1DForOutWhenUnconnected=off
  dataValid : Outport  Port=2  VectorParamsAs1DForOutWhenUnconnected=off
  preambleValid : Outport  Port=3  VectorParamsAs1DForOutWhenUnconnected=off
  wires:
  OR/1 -> FFTValid/1
  dataValidGen/1(y) -> dataValid/1, OR/2
  PreambleValidGen/1(y) -> dataValidGen/1(enb), OR/1, preambleValid/1
  validIn/1 -> PreambleValidGen/1(ValidIn), dataValidGen/2(enb1)

== system lib_ofdmrx/OFDMRx/Synchronisation/Delay ==
  note: Delay coarse timing point from middle of L-STF
      | to beginning of 1st repetition of L-LTF
  data : Inport
  strobe : Inport  Port=2
  Delay3 : Delay  DelayLength=108  InputProcessing=Columns as channels (frame based)
  dataOut : Outport
  strobeOut : Outport  Port=2
  wires:
  data/1 -> dataOut/1
  Delay3/1 -> strobeOut/1
  strobe/1 -> Delay3/1

== system lib_ofdmrx/OFDMRx/Synchronisation/FrameDetect ==
  note: The frame is detected when the timing metric exceeds the threshold for 30 successive samples. This
      | corresponds to the coarse timing point, which should occur in the middle of the L-STF.
  leftIn : Inport
  rightIn : Inport  Port=2
  phaseIn : Inport  Port=3
  Compare To Constant : simulink/Logic and Bit Operations/Compare To Constant  relop===  const=29  OutDataTypeStr=boolean
  Delay{,2..4} (4 alike) : Delay  DelayLength=1
  HDL Counter : hdlsllib/Sources/HDL Counter  CountType=Count limited  CountInit=0  CountStep=1  CountMax=29  CountFromType=Initial value  CountFrom=0  CountResetPort=on  CountLoadPort=off  CountEnbPort=on  CountDirPort=off  CountDataType=Unsigned  CountWordLen=5  CountFracLen=0  CountSampTime=1
  Logical Operator : Logic  Operator=OR  IconShape=distinctive  AllPortsSameDT=off  OutDataTypeStr=boolean
  Logical Operator1 : Logic  Operator=NOT  IconShape=distinctive  AllPortsSameDT=off  OutDataTypeStr=boolean
  Relational Operator : RelationalOperator  Operator=>  OutDataTypeStr=boolean  RndMeth=Simplest
  RsingEdge : Subsystem
  frameDet : Outport  VectorParamsAs1DForOutWhenUnconnected=off
  phaseOut : Outport  Port=2  VectorParamsAs1DForOutWhenUnconnected=off
  wires:
  Delay3/1 -> Relational Operator/2
  Relational Operator/1 -> HDL Counter/2, Logical Operator1/1
  Logical Operator1/1 -> Logical Operator/2
  rightIn/1 -> Delay3/1
  HDL Counter/1 -> Compare To Constant/1
  Compare To Constant/1 -> RsingEdge/1(In1), Logical Operator/1
  Logical Operator/1 -> HDL Counter/1
  phaseIn/1 -> Delay4/1
  leftIn/1 -> Delay2/1
  Delay/1 -> phaseOut/1
  RsingEdge/1(Out1) -> frameDet/1
  Delay2/1 -> Relational Operator/1
  Delay4/1 -> Delay/1

== system lib_ofdmrx/OFDMRx/Synchronisation/SchmidlCoxMetric  ==
  note: The Schmidl & Cox timing metric is used for frame detection. The timing metric, M(d), is compared to a threshold
      | to determine if a frame is present. In order to avoid division, we re-arrange the timing metric as |P(d)|^2 > (R(d))^2 x thresh.
      | The phase of the averaged autocorrelation is also determined for Carrier Frequency Offset (CFO) estimation purposes.
  note: |P(d)|^2
  note: (R(d))^2 x thresh
  dataIn : Inport
  Abs2 : Subsystem
  AutoCorr : Subsystem
  CIC_ma : Subsystem
  CIC_ma1 : Subsystem
  Delay : Delay  DelayLength=14
  Delay2 : Delay
  MagPhase : Subsystem
  Sq : Subsystem
  Sq1 : Subsystem
  ThreshMult : Subsystem
  left : Outport  VectorParamsAs1DForOutWhenUnconnected=off
  right : Outport  Port=2  VectorParamsAs1DForOutWhenUnconnected=off
  phase : Outport  Port=3  VectorParamsAs1DForOutWhenUnconnected=off
  wires:
  Sq/1(Out1) -> left/1
  ThreshMult/1(Out1) -> right/1
  Sq1/1(Out1) -> ThreshMult/1(In1)
  Delay/1 -> Sq1/1(In1)
  CIC_ma1/1(Out1) -> Delay/1
  dataIn/1 -> AutoCorr/1(AcorrIn), Abs2/1(Abs2In)
  Abs2/1(Abs2Out) -> CIC_ma1/1(In1)
  MagPhase/2(Mag) -> Sq/1(In1)
  AutoCorr/1(AcorrOut) -> CIC_ma/1(In1)
  CIC_ma/1(Out1) -> MagPhase/1(dataIn)
  Delay2/1 -> phase/1
  MagPhase/1(Phase) -> Delay2/1

== system lib_ofdmrx/OFDMRx/ChannelEstEq/ChannelEstimate/ChanEst ==
  note: 2nd half
  note: 1st half
  note: Read out frequency domain LTS
      | when preamble valid is HIGH and
      | use this to obtain channel estimate.
  note: Store conjugate as this is used in the
      | equaliser.
  ChanEstIn : Inport
  PreambValidIn : Inport  Port=2
  Delay : Delay  DelayLength=64
  Delay{1..7} (7 alike) : Delay  DelayLength=1
  Gain : Gain  Gain=0.5  OutDataTypeStr=fixdt(1,17,14)
  HDL Counter : hdlsllib/Sources/HDL Counter  CountType=Count limited  CountInit=0  CountStep=1  CountMax=63  CountFromType=Initial value  CountFrom=0  CountResetPort=off  CountLoadPort=off  CountEnbPort=on  CountDirPort=off  CountDataType=Unsigned  CountWordLen=6  CountFracLen=0  CountSampTime=1
  InvLLTF : Lookup_n-D  NumberOfTableDimensions=1  BreakpointsForDimension1=0:63  IndexSearchMethod=Evenly spaced points  Table=fftshift(LTSfreq)  TableDataTypeStr=fixdt(1,16,0)  InterpMethod=Flat  ExtrapMethod=Clip  DiagnosticForOutOfRangeInput=Error  UseLastTableValue=on  InternalRulePriority=Speed  OutDataTypeStr=fixdt(1,16,0)  RndMeth=Simplest  InputSameDT=on
  Math Function : Math  Operator=conj  SignedPower=on  SaturateOnIntegerOverflow=on
  Product : Product  OutDataTypeStr=fixdt(1,16,14)
  Subtract : Sum
  ChEstOut : Outport  VectorParamsAs1DForOutWhenUnconnected=off
  wires:
  Subtract/1 -> Gain/1
  Delay3/1 -> ChEstOut/1
  Delay2/1 -> HDL Counter/1
  Delay1/1 -> Delay4/1
  PreambValidIn/1 -> Delay2/1
  ChanEstIn/1 -> Delay1/1
  Math Function/1 -> Delay3/1
  Delay/1 -> Subtract/1
  Product/1 -> Delay6/1
  Gain/1 -> Delay7/1
  HDL Counter/1 -> InvLLTF/1
  Delay4/1 -> Product/1
  InvLLTF/1 -> Delay5/1
  Delay5/1 -> Product/2
  Delay6/1 -> Delay/1, Subtract/2
  Delay7/1 -> Math Function/1

== system lib_ofdmrx/OFDMRx/ChannelEstEq/ChannelEstimate/WriteEnbAddrGen ==
  In1 : Inport
  AND : Logic  IconShape=distinctive  AllPortsSameDT=off  OutDataTypeStr=boolean
  Compare To Constant : simulink/Logic and Bit Operations/Compare To Constant  relop=>=  const=64  OutDataTypeStr=boolean
  Compare To Constant1 : simulink/Logic and Bit Operations/Compare To Constant  relop=<=  const=127  OutDataTypeStr=boolean
  HDL Counter1 : hdlsllib/Sources/HDL Counter  CountType=Count limited  CountInit=0  CountStep=1  CountMax=63  CountFromType=Initial value  CountFrom=0  CountResetPort=off  CountLoadPort=off  CountEnbPort=on  CountDirPort=off  CountDataType=Unsigned  CountWordLen=6  CountFracLen=0  CountSampTime=1
  HDL Counter2 : hdlsllib/Sources/HDL Counter  CountType=Count limited  CountInit=0  CountStep=1  CountMax=127  CountFromType=Initial value  CountFrom=0  CountResetPort=off  CountLoadPort=off  CountEnbPort=on  CountDirPort=off  CountDataType=Unsigned  CountWordLen=7  CountFracLen=0  CountSampTime=1
  Out1 : Outport  VectorParamsAs1DForOutWhenUnconnected=off
  Out2 : Outport  Port=2  VectorParamsAs1DForOutWhenUnconnected=off
  wires:
  Compare To Constant1/1 -> AND/2
  Compare To Constant/1 -> AND/1
  HDL Counter1/1 -> Out1/1
  AND/1 -> HDL Counter1/1, Out2/1
  HDL Counter2/1 -> Compare To Constant1/1, Compare To Constant/1
  In1/1 -> HDL Counter2/1

== system lib_ofdmrx/OFDMRx/ChannelEstEq/Equalise/Abs2 ==
  ChEstIn : Inport
  Add : Sum  OutDataTypeStr=fixdt(0,16,14)
  Complex to Real-Imag : ComplexToRealImag
  Delay{,1..4} (5 alike) : Delay  DelayLength=1
  Product : Product
  Product1 : Product
  Out1 : Outport  VectorParamsAs1DForOutWhenUnconnected=off
  wires:
  Delay4/1 -> Out1/1
  Add/1 -> Delay4/1
  Complex to Real-Imag/1 -> Delay/1
  ChEstIn/1 -> Complex to Real-Imag/1
  Product/1 -> Delay2/1
  Product1/1 -> Delay3/1
  Complex to Real-Imag/2 -> Delay1/1
  Delay/1 -> Product/1, Product/2
  Delay1/1 -> Product1/2, Product1/1
  Delay2/1 -> Add/1
  Delay3/1 -> Add/2

== system lib_ofdmrx/OFDMRx/ChannelEstEq/Equalise/Complex Mult ==
  In1 : Inport
  In2 : Inport  Port=2
  Delay4 : Delay  DelayLength=1
  Delay5 : Delay  DelayLength=1
  Delay7 : Delay
  Product1 : Product  OutDataTypeStr=fixdt(1,18,15)
  Out1 : Outport
  wires:
  In2/1 -> Delay5/1
  Delay7/1 -> Out1/1
  Delay5/1 -> Product1/2
  In1/1 -> Delay4/1
  Delay4/1 -> Product1/1
  Product1/1 -> Delay7/1

== system lib_ofdmrx/OFDMRx/ChannelEstEq/Equalise/Divide ==
  In1 : Inport
  In2 : Inport  Port=2
  Delay1 : Delay  DelayLength=1
  Delay2 : Delay  DelayLength=1
  Delay8 : Delay  DelayLength=1
  Product2 : Product  OutDataTypeStr=fixdt(1,18,15)
  Reciprocal : Product  Inputs=/  OutDataTypeStr=fixdt(0,25,15)  RndMeth=Zero  SaturateOnIntegerOverflow=on
  dataOutEq : Outport
  wires:
  Delay2/1 -> dataOutEq/1
  Product2/1 -> Delay2/1
  Delay1/1 -> Product2/2
  Delay8/1 -> Product2/1
  In1/1 -> Delay8/1
  In2/1 -> Reciprocal/1
  Reciprocal/1 -> Delay1/1

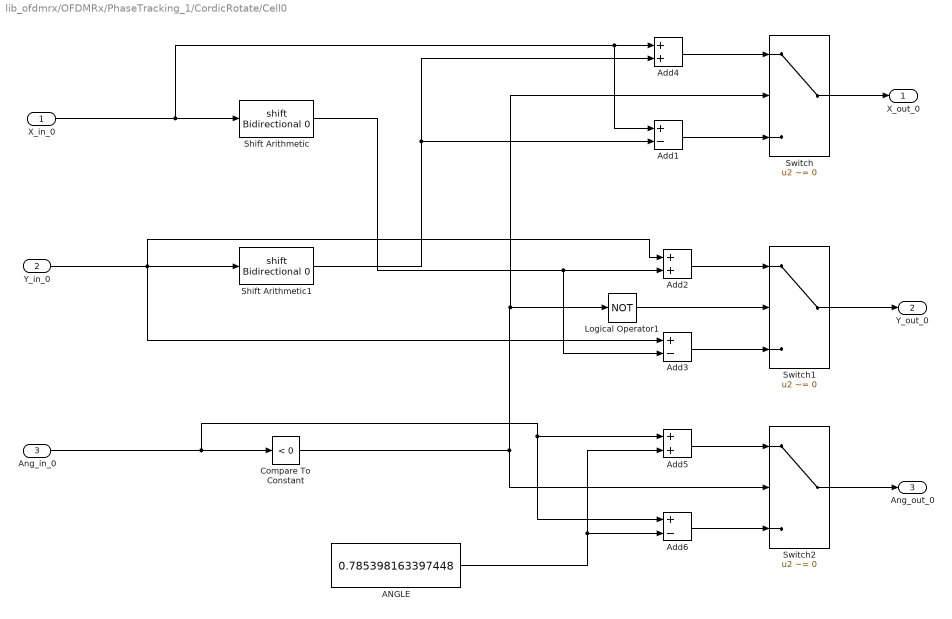
== system lib_ofdmrx/OFDMRx/PhaseTracking_1/CordicRotate/Cell0 ==
  X_in_0 : Inport
  Y_in_0 : Inport  Port=2
  Ang_in_0 : Inport  Port=3
  ANGLE : Constant  Value=0.785398163397448  VectorParams1D=off  OutDataTypeStr=fixdt(1,23,20)  SampleTime=1/fs
  Add1 : Sum  Inputs=+-  OutDataTypeStr=fixdt(1,21,15)
  Add2 : Sum  OutDataTypeStr=fixdt(1,21,15)
  Add3 : Sum  Inputs=+-  OutDataTypeStr=fixdt(1,21,15)
  Add4 : Sum  OutDataTypeStr=fixdt(1,21,15)
  Add5 : Sum  OutDataTypeStr=fixdt(1,23,20)
  Add6 : Sum  Inputs=+-  OutDataTypeStr=fixdt(1,23,20)
  Compare To Constant : simulink/Logic and Bit Operations/Compare To Constant  relop=<  const=0  OutDataTypeStr=boolean
  Logical Operator1 : Logic  Operator=NOT  IconShape=distinctive  AllPortsSameDT=off  OutDataTypeStr=boolean
  Shift Arithmetic : ArithShift
  Shift Arithmetic1 : ArithShift
  Switch : Switch  Criteria=u2 ~= 0
  Switch1 : Switch  Criteria=u2 ~= 0
  Switch2 : Switch  Criteria=u2 ~= 0
  X_out_0 : Outport  VectorParamsAs1DForOutWhenUnconnected=off
  Y_out_0 : Outport  Port=2  VectorParamsAs1DForOutWhenUnconnected=off
  Ang_out_0 : Outport  Port=3  VectorParamsAs1DForOutWhenUnconnected=off
  wires:
  Add4/1 -> Switch/1
  Add1/1 -> Switch/3
  Add3/1 -> Switch1/3
  Add2/1 -> Switch1/1
  Switch/1 -> X_out_0/1
  Switch1/1 -> Y_out_0/1
  Add6/1 -> Switch2/3
  Add5/1 -> Switch2/1
  Switch2/1 -> Ang_out_0/1
  X_in_0/1 -> Shift Arithmetic/1, Add1/1, Add4/1
  Y_in_0/1 -> Shift Arithmetic1/1, Add3/1, Add2/1
  Ang_in_0/1 -> Add6/1, Add5/1, Compare To Constant/1
  Compare To Constant/1 -> Logical Operator1/1, Switch/2, Switch2/2
  Shift Arithmetic1/1 -> Add1/2, Add4/2
  Shift Arithmetic/1 -> Add3/2, Add2/2
  Logical Operator1/1 -> Switch1/2
  ANGLE/1 -> Add6/2, Add5/2

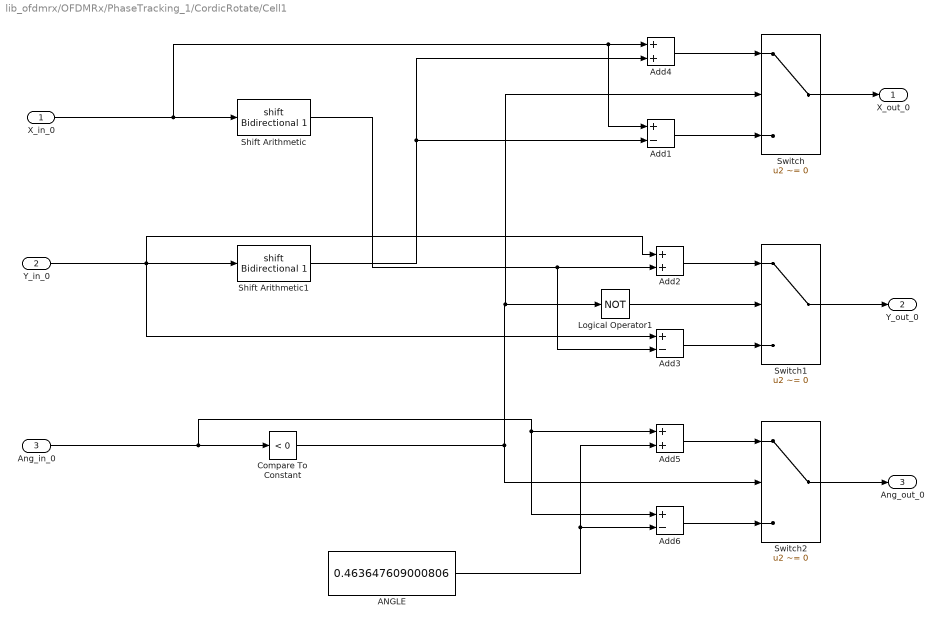
== system lib_ofdmrx/OFDMRx/PhaseTracking_1/CordicRotate/Cell1 ==
  X_in_0 : Inport
  Y_in_0 : Inport  Port=2
  Ang_in_0 : Inport  Port=3
  ANGLE : Constant  Value=0.463647609000806  VectorParams1D=off  OutDataTypeStr=fixdt(1,23,20)  SampleTime=1/fs
  Add1 : Sum  Inputs=+-  OutDataTypeStr=fixdt(1,21,15)
  Add2 : Sum  OutDataTypeStr=fixdt(1,21,15)
  Add3 : Sum  Inputs=+-  OutDataTypeStr=fixdt(1,21,15)
  Add4 : Sum  OutDataTypeStr=fixdt(1,21,15)
  Add5 : Sum  OutDataTypeStr=fixdt(1,23,20)
  Add6 : Sum  Inputs=+-  OutDataTypeStr=fixdt(1,23,20)
  Compare To Constant : simulink/Logic and Bit Operations/Compare To Constant  relop=<  const=0  OutDataTypeStr=boolean
  Logical Operator1 : Logic  Operator=NOT  IconShape=distinctive  AllPortsSameDT=off  OutDataTypeStr=boolean
  Shift Arithmetic : ArithShift  BitShiftNumber=1
  Shift Arithmetic1 : ArithShift  BitShiftNumber=1
  Switch : Switch  Criteria=u2 ~= 0
  Switch1 : Switch  Criteria=u2 ~= 0
  Switch2 : Switch  Criteria=u2 ~= 0
  X_out_0 : Outport  VectorParamsAs1DForOutWhenUnconnected=off
  Y_out_0 : Outport  Port=2  VectorParamsAs1DForOutWhenUnconnected=off
  Ang_out_0 : Outport  Port=3  VectorParamsAs1DForOutWhenUnconnected=off
  wires:
  ANGLE/1 -> Add5/2, Add6/2
  Logical Operator1/1 -> Switch1/2
  Shift Arithmetic/1 -> Add2/2, Add3/2
  Shift Arithmetic1/1 -> Add4/2, Add1/2
  Compare To Constant/1 -> Switch2/2, Switch/2, Logical Operator1/1
  Ang_in_0/1 -> Compare To Constant/1, Add5/1, Add6/1
  Y_in_0/1 -> Add2/1, Add3/1, Shift Arithmetic1/1
  X_in_0/1 -> Add4/1, Add1/1, Shift Arithmetic/1
  Switch2/1 -> Ang_out_0/1
  Add5/1 -> Switch2/1
  Add6/1 -> Switch2/3
  Switch1/1 -> Y_out_0/1
  Switch/1 -> X_out_0/1
  Add2/1 -> Switch1/1
  Add3/1 -> Switch1/3
  Add1/1 -> Switch/3
  Add4/1 -> Switch/1

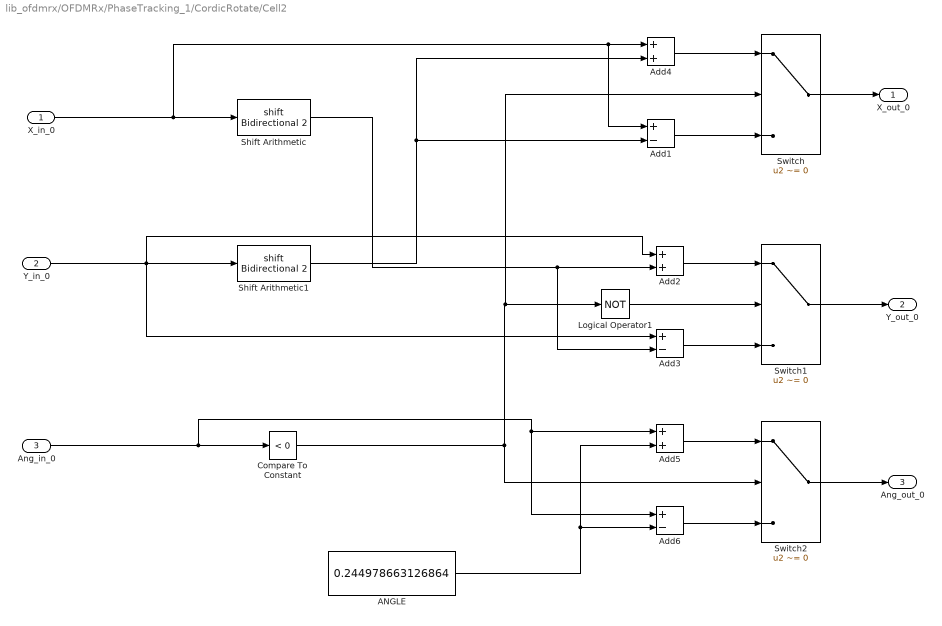
== system lib_ofdmrx/OFDMRx/PhaseTracking_1/CordicRotate/Cell2 ==
  X_in_0 : Inport
  Y_in_0 : Inport  Port=2
  Ang_in_0 : Inport  Port=3
  ANGLE : Constant  Value=0.244978663126864  VectorParams1D=off  OutDataTypeStr=fixdt(1,23,20)  SampleTime=1/fs
  Add1 : Sum  Inputs=+-  OutDataTypeStr=fixdt(1,21,15)
  Add2 : Sum  OutDataTypeStr=fixdt(1,21,15)
  Add3 : Sum  Inputs=+-  OutDataTypeStr=fixdt(1,21,15)
  Add4 : Sum  OutDataTypeStr=fixdt(1,21,15)
  Add5 : Sum  OutDataTypeStr=fixdt(1,23,20)
  Add6 : Sum  Inputs=+-  OutDataTypeStr=fixdt(1,23,20)
  Compare To Constant : simulink/Logic and Bit Operations/Compare To Constant  relop=<  const=0  OutDataTypeStr=boolean
  Logical Operator1 : Logic  Operator=NOT  IconShape=distinctive  AllPortsSameDT=off  OutDataTypeStr=boolean
  Shift Arithmetic : ArithShift  BitShiftNumber=2
  Shift Arithmetic1 : ArithShift  BitShiftNumber=2
  Switch : Switch  Criteria=u2 ~= 0
  Switch1 : Switch  Criteria=u2 ~= 0
  Switch2 : Switch  Criteria=u2 ~= 0
  X_out_0 : Outport  VectorParamsAs1DForOutWhenUnconnected=off
  Y_out_0 : Outport  Port=2  VectorParamsAs1DForOutWhenUnconnected=off
  Ang_out_0 : Outport  Port=3  VectorParamsAs1DForOutWhenUnconnected=off
  wires:
  Add4/1 -> Switch/1
  Add1/1 -> Switch/3
  Add3/1 -> Switch1/3
  Add2/1 -> Switch1/1
  Switch/1 -> X_out_0/1
  Switch1/1 -> Y_out_0/1
  Add6/1 -> Switch2/3
  Add5/1 -> Switch2/1
  Switch2/1 -> Ang_out_0/1
  X_in_0/1 -> Shift Arithmetic/1, Add1/1, Add4/1
  Y_in_0/1 -> Shift Arithmetic1/1, Add3/1, Add2/1
  Ang_in_0/1 -> Add6/1, Add5/1, Compare To Constant/1
  Compare To Constant/1 -> Logical Operator1/1, Switch/2, Switch2/2
  Shift Arithmetic1/1 -> Add1/2, Add4/2
  Shift Arithmetic/1 -> Add3/2, Add2/2
  Logical Operator1/1 -> Switch1/2
  ANGLE/1 -> Add6/2, Add5/2

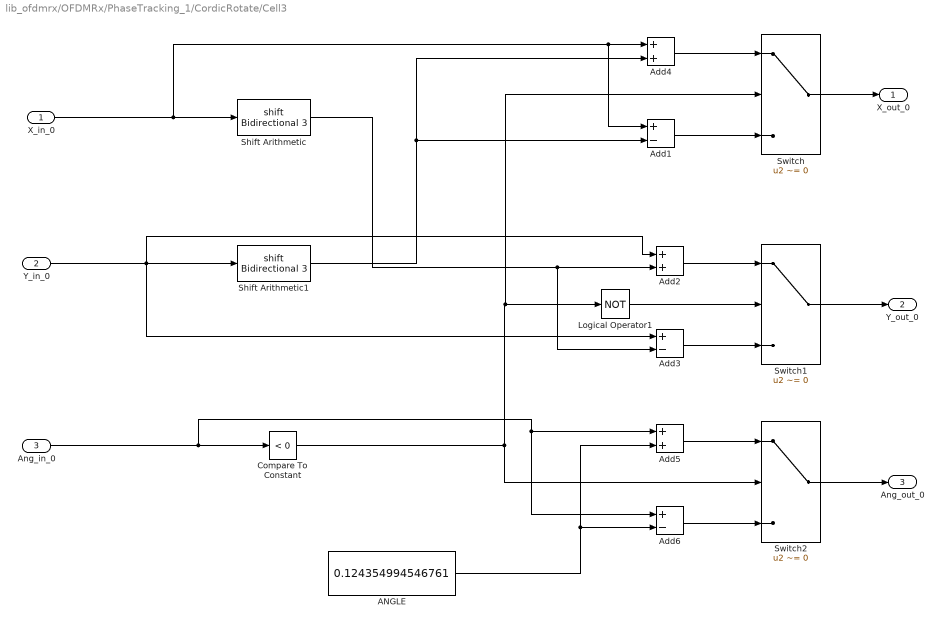
== system lib_ofdmrx/OFDMRx/PhaseTracking_1/CordicRotate/Cell3 ==
  X_in_0 : Inport
  Y_in_0 : Inport  Port=2
  Ang_in_0 : Inport  Port=3
  ANGLE : Constant  Value=0.124354994546761  VectorParams1D=off  OutDataTypeStr=fixdt(1,23,20)  SampleTime=1/fs
  Add1 : Sum  Inputs=+-  OutDataTypeStr=fixdt(1,21,15)
  Add2 : Sum  OutDataTypeStr=fixdt(1,21,15)
  Add3 : Sum  Inputs=+-  OutDataTypeStr=fixdt(1,21,15)
  Add4 : Sum  OutDataTypeStr=fixdt(1,21,15)
  Add5 : Sum  OutDataTypeStr=fixdt(1,23,20)
  Add6 : Sum  Inputs=+-  OutDataTypeStr=fixdt(1,23,20)
  Compare To Constant : simulink/Logic and Bit Operations/Compare To Constant  relop=<  const=0  OutDataTypeStr=boolean
  Logical Operator1 : Logic  Operator=NOT  IconShape=distinctive  AllPortsSameDT=off  OutDataTypeStr=boolean
  Shift Arithmetic : ArithShift  BitShiftNumber=3
  Shift Arithmetic1 : ArithShift  BitShiftNumber=3
  Switch : Switch  Criteria=u2 ~= 0
  Switch1 : Switch  Criteria=u2 ~= 0
  Switch2 : Switch  Criteria=u2 ~= 0
  X_out_0 : Outport  VectorParamsAs1DForOutWhenUnconnected=off
  Y_out_0 : Outport  Port=2  VectorParamsAs1DForOutWhenUnconnected=off
  Ang_out_0 : Outport  Port=3  VectorParamsAs1DForOutWhenUnconnected=off
  wires:
  ANGLE/1 -> Add5/2, Add6/2
  Logical Operator1/1 -> Switch1/2
  Shift Arithmetic/1 -> Add2/2, Add3/2
  Shift Arithmetic1/1 -> Add4/2, Add1/2
  Compare To Constant/1 -> Switch2/2, Switch/2, Logical Operator1/1
  Ang_in_0/1 -> Compare To Constant/1, Add5/1, Add6/1
  Y_in_0/1 -> Add2/1, Add3/1, Shift Arithmetic1/1
  X_in_0/1 -> Add4/1, Add1/1, Shift Arithmetic/1
  Switch2/1 -> Ang_out_0/1
  Add5/1 -> Switch2/1
  Add6/1 -> Switch2/3
  Switch1/1 -> Y_out_0/1
  Switch/1 -> X_out_0/1
  Add2/1 -> Switch1/1
  Add3/1 -> Switch1/3
  Add1/1 -> Switch/3
  Add4/1 -> Switch/1
